simulink model "silly_test_name"  (R2018a)
settings: Solver=FixedStepAuto  StartTime=0.0  StopTime=10.0  FixedStep=1e-3  RelTol=1e-3
libraries: sl_kafka_lib x2
settings Model: Creator=asolland  LastModifiedBy=asolland
settings DataIOCC: ReturnWorkspaceOutputs=on
settings OptimizationCC: DefaultParameterBehavior=Inlined  EnhancedBackFolding=on  PassReuseOutputArgsAs=Individual arguments  ZeroExternalMemoryAtStartup=off  ZeroInternalMemoryAtStartup=off  OptimizeBlockOrder=speed  DifferentSizesBufferReuse=on  OptimizationCustomize=off
settings DebuggingCC: ParameterTunabilityLossMsg=error
settings HardwareCC: ProdBitPerLong=64  ProdHWDeviceType=Intel->x86-64 (Linux 64)
settings SFSimCC: SimUseLocalCustomCode=on  MATLABDynamicMemAlloc=off
settings RTWCC: Description=Kafka Target  SystemTargetFile=kafkatarget.tlc  TemplateMakefile=ert_default_tmf  GenerateReport=on  RTWUseLocalCustomCode=on  IncludeHyperlinkInReport=on  LaunchReport=on  GenerateTraceInfo=on  GenerateTraceReport=on  GenerateTraceReportSl=on  GenerateTraceReportSf=on  GenerateTraceReportEml=on
settings CodeAppCC: ForceParamTrailComments=on  IgnoreCustomStorageClasses=off  OperatorAnnotations=on  SimulinkDataObjDesc=on  SFDataObjDesc=on  InsertBlockDesc=on
settings STFCustomTargetCC: TargetLangStandard=C99 (ISO)  MultiwordLength=256  GenerateSampleERTMain=on  CombineOutputUpdateFcns=on  ERTCustomFileBanners=on  SupportContinuousTime=off  SupportNonInlinedSFcns=off  RemoveResetFunc=on  MATLABClassNameForMDSCustomization=Simulink.SoftwareTarget.ERTCustomization  GRTInterface=off  UseToolchainInfoCompliant=on  SystemTargetFile=kafkatarget.tlc
settings ERTTargetCC: TargetLangStandard=C99 (ISO)  GenerateSampleERTMain=on  ParMdlRefBuildCompliant=off  CompOptLevelCompliant=off  ConcurrentExecutionCompliant=off  ModelStepFunctionPrototypeControlCompliant=off  CPPClassGenCompliant=off  InlinedParameterPlacement=NonHierarchical  ERTCustomFileTemplate=kafkatarget_process.tlc

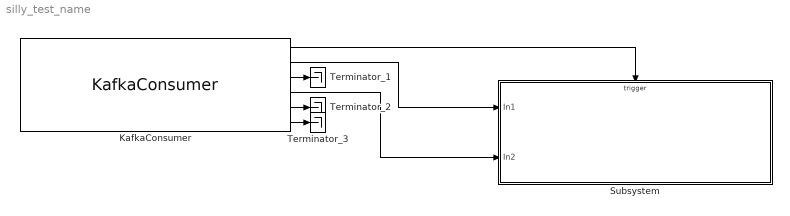
== system silly_test_name ==
  KafkaConsumer : sl_kafka_lib/KafkaConsumer  sfpBrokers='localhost:9092'  sfpTopic='sl_in'  sfpGroup='abc'  sfpMsgLen=128  sfpKeyLen=32  sfpOutputTimestamp=on  sfpTS=.1  sfpConf=|  sfpTopicConf=compression.level=-1
      | client.id=sl_kafka_consumer
      | message.copy.max.bytes=65535
      settings: SourceProductName=Kafka Library
  Subsystem : Subsystem
  Terminator_1 : Terminator
  Terminator_2 : Terminator
  Terminator_3 : Terminator
  wires:
  KafkaConsumer/2 -> Subsystem/1(In1)
  KafkaConsumer/4 -> Subsystem/2(In2)
  KafkaConsumer/1 -> Subsystem/Trigger
  KafkaConsumer/3 -> Terminator_1/1
  KafkaConsumer/5 -> Terminator_2/1
  KafkaConsumer/6 -> Terminator_3/1

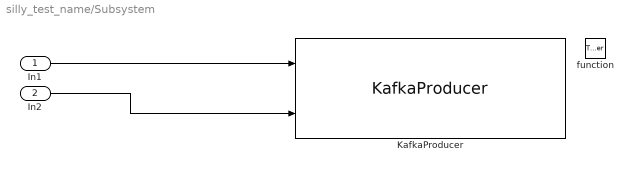
== system silly_test_name/Subsystem ==
  In1 : Inport
  In2 : Inport  Port=2
  function : TriggerPort  TriggerType=function-call  VariantControl=Variant
  KafkaProducer : sl_kafka_lib/KafkaProducer  sfpBrokers='localhost:9092'  sfpTopic='sl_out'  sfpKeyAsInput=on  sfpKeyAsInputLen=32  sfpKey='mykey'  sfpMsgLen=128  sfpTS=-1  sfpConf=|  sfpTopicConf=compression.level=-1
      | client.id=sl_kafka_producer
      | message.copy.max.bytes=65535
      settings: SourceProductName=Kafka Library
  wires:
  In2/1 -> KafkaProducer/2
  In1/1 -> KafkaProducer/1
